simulink model "Exercise_1"  (R2024b)
settings: Solver=VariableStepAuto  StartTime=0.0  StopTime=10.0  RelTol=1e-3
libraries: dspfdesign x2
settings Model: Creator=HP  LastModifiedBy=HP

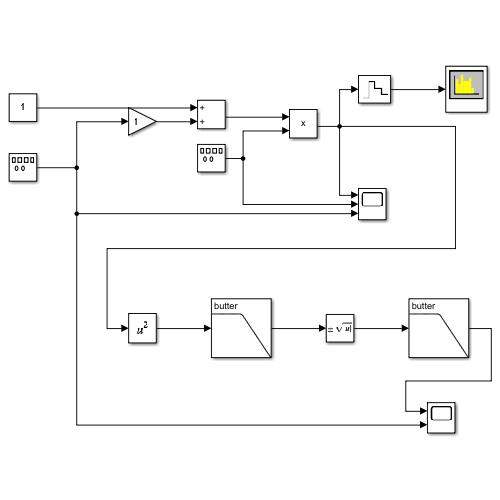
[thumbnail: Simulink's stored preview of the top-level diagram]
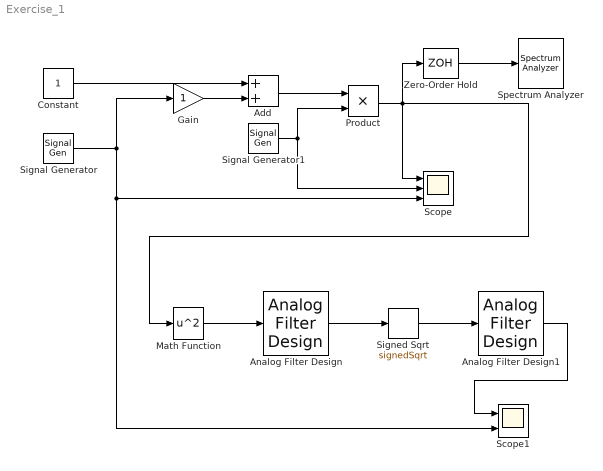
== system Exercise_1 ==
  Add : Sum
  Analog Filter Design : dspfdesign/Analog Filter Design  method=Butterworth  filttype=Lowpass  N=8  Wlo=30  Whi=80  Rp=2  Rs=40
  Analog Filter Design1 : dspfdesign/Analog Filter Design  method=Butterworth  filttype=Lowpass  N=8  Wlo=30  Whi=80  Rp=2  Rs=40
  Constant : Constant
  Gain : Gain
  Math Function : Math  Operator=square
  Product : Product
  Scope : Scope  NumInputPorts=3
  Scope1 : Scope  NumInputPorts=2
  Signal Generator : SignalGenerator  Frequency=2000
  Signal Generator1 : SignalGenerator  Amplitude=2  Frequency=20000
  Signed Sqrt : Sqrt  Operator=signedSqrt
  Spectrum Analyzer : SpectrumAnalyzer  WindowPosition=[1.000000,41.000000,1536.000000,800.000000,]  ScopeFrameLocation=window  SampleRate=44.1e3  PlotAsTwoSidedSpectrum=off  FrequencyScale=Log  WindowInvariantSamplesPerUpdate=on  FrequencySpan=Start and stop frequencies  StartFrequency=20  StopFrequency=20e3  YLimits=[-146.51259882,45.80725898]
  Zero-Order Hold : ZeroOrderHold  SampleTime=-1
  wires:
  Zero-Order Hold/1 -> Spectrum Analyzer/1
  Constant/1 -> Add/1
  Add/1 -> Product/1
  Signal Generator/1 -> Scope/3, Scope1/2, Gain/1
  Signal Generator1/1 -> Product/2, Scope/2
  Analog Filter Design/1 -> Signed Sqrt/1
  Signed Sqrt/1 -> Analog Filter Design1/1
  Analog Filter Design1/1 -> Scope1/1
  Math Function/1 -> Analog Filter Design/1
  Product/1 -> Zero-Order Hold/1, Scope/1, Math Function/1
  Gain/1 -> Add/2
